simulink library "control_allocation_lib"  (R2018b)
settings: Solver=VariableStepAuto  StartTime=0.0  StopTime=10.0  RelTol=1e-3
undefined symbols (not defined in the file or in its folder): ca
libraries: $bdroot x1
settings Model: Creator=Ybeyer  LastModifiedBy=yannic
settings DebuggingCC: LibraryContextMissingDiagnostic=none
settings SFSimCC: SimUseLocalCustomCode=off
settings RTWCC: RTWUseLocalCustomCode=off
settings CodeAppCC: StateflowObjectComments=on

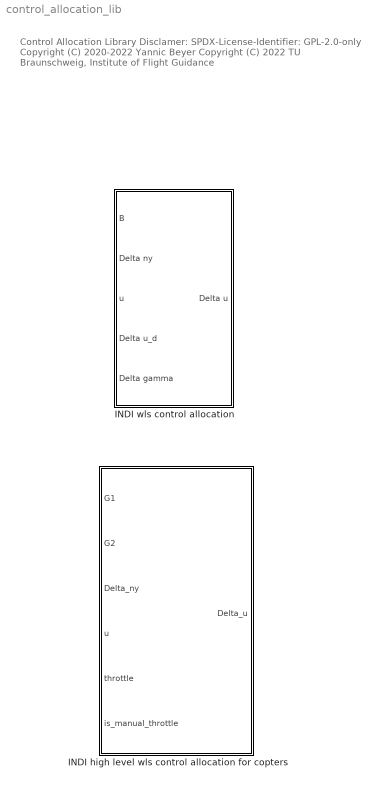
== system control_allocation_lib ==
  note: Control Allocation Library
      |
      | Disclamer:
      | SPDX-License-Identifier: GPL-2.0-only
      |
      | Copyright (C) 2020-2022 Yannic Beyer
      | Copyright (C) 2022 TU Braunschweig, Institute of Flight Guidance
  INDI high level wls control allocation for copters : Subsystem  mask{ca=ca}
      mask prompts: ca "control allocation parameters struct"
      mask DialogControl DescGroupVar Prompt: INDI high level control allocation
      mask DialogControl DescTextVar Prompt: It wraps the INDI control allocation block and adds some high level usability features.
      mask DialogControl Control2 Prompt: This block makes manual throttle control possible. Moreover, it not only considers the control effectiveness G1 but also the effectiveness of the control input derivative G2 [1].
      mask DialogControl Control3 Prompt: [1] Smeur, E. J., Chu, Q., & de Croon, G. C. (2016). Adaptive incremental nonlinear dynamic inversion for attitude control of micro air vehicles. Journal of Guidance, Control, and Dynamics, 39(3), 450-461.
      mask DialogControl Control4 Prompt: To load a control allocation parameters struct, see controlAllocationWlsLoadParams
  INDI wls control allocation : Subsystem  mask{ca=ca}
      mask prompts: ca "control allocation parameters struct"
      mask DialogControl DescGroupVar Prompt: INDI control allocation
      mask DialogControl DescTextVar Prompt: Solve wls control allocation algorithm for INDI.
      mask DialogControl Control2 Prompt: The control allocation algorithm is adjusted to INDI according to
      mask DialogControl Control3 Prompt: Smeur, E., Höppener, D., & Wagter, C. D. (2017). Prioritized Control Allocation for Quadrotors Subject to Saturation, In H. D. P. J.-M. Moschetta, G. Hattenberger (Ed.), International Micro Air Vehicle Conference and Flight Competition 2017 (pp. 37-43). Toulouse, France.
      mask DialogControl Control4 Prompt: To load a control allocation parameters struct, see controlAllocationWlsLoadParams

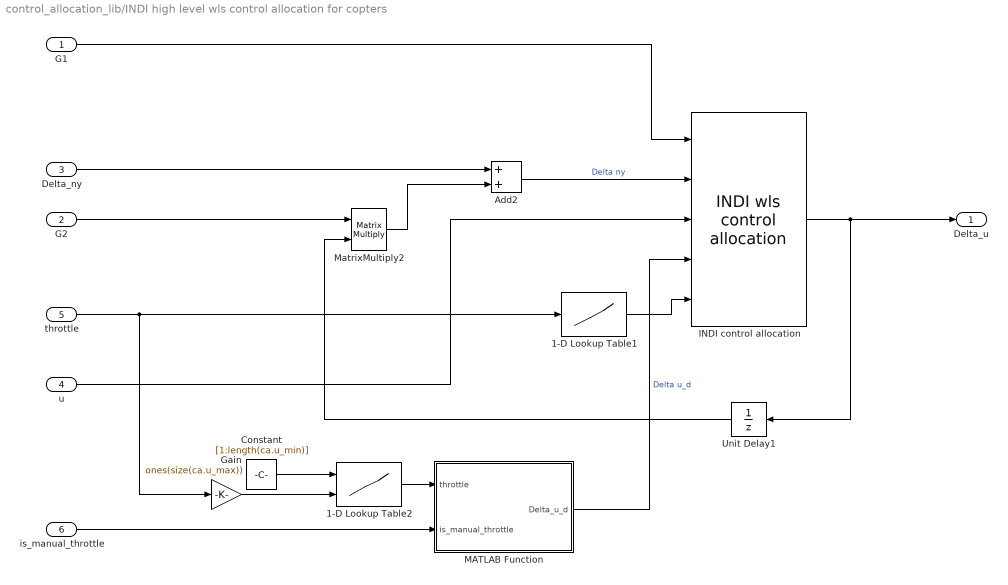
== system control_allocation_lib/INDI high level wls control allocation for copters ==
  G1 : Inport
  G2 : Inport  Port=2
  Delta_ny : Inport  Port=3
  u : Inport  Port=4
  throttle : Inport  Port=5
  is_manual_throttle : Inport  Port=6
  1-D Lookup Table1 : Lookup_n-D  NumberOfTableDimensions=1  BreakpointsForDimension1=[0,0.1,0.2,1]  Table=[-0.99999999*ca.gamma*[1,1],0,0]  InternalRulePriority=Speed  RndMeth=Simplest  InputSameDT=on
  1-D Lookup Table2 : Lookup_n-D  BreakpointsForDimension1=[1:length(ca.u_min)]'  BreakpointsForDimension2=[0,1]  Table=[ca.u_min,ca.u_max]  ExtrapMethod=Clip  InternalRulePriority=Speed  RndMeth=Simplest  InputSameDT=on
  Add2 : Sum
  Constant : Constant  Value=[1:length(ca.u_min)]  OutDataTypeStr=Inherit: Inherit via back propagation
  Gain : Gain  Gain=ones(size(ca.u_max))
  INDI control allocation : $bdroot/INDI wls control allocation  ca=ca
  MATLAB Function : MATLAB Function  TreatAsAtomicUnit=on
  MatrixMultiply2 : Product  Multiplication=Matrix(*)
  Unit Delay1 : UnitDelay  SampleTime=-1
  Delta_u : Outport
  wires:
  throttle/1 -> Gain/1, 1-D Lookup Table1/1
  G2/1 -> MatrixMultiply2/1
  MatrixMultiply2/1 -> Add2/2
  G1/1 -> INDI control allocation/1
  Add2/1 -> INDI control allocation/2  "Delta ny"
  u/1 -> INDI control allocation/3
  INDI control allocation/1 -> Delta_u/1, Unit Delay1/1
  1-D Lookup Table1/1 -> INDI control allocation/5
  Delta_ny/1 -> Add2/1
  Unit Delay1/1 -> MatrixMultiply2/2
  MATLAB Function/1(Delta_u_d) -> INDI control allocation/4  "Delta u_d"
  is_manual_throttle/1 -> MATLAB Function/2(is_manual_throttle)
  1-D Lookup Table2/1 -> MATLAB Function/1(throttle)
  Gain/1 -> 1-D Lookup Table2/2
  Constant/1 -> 1-D Lookup Table2/1

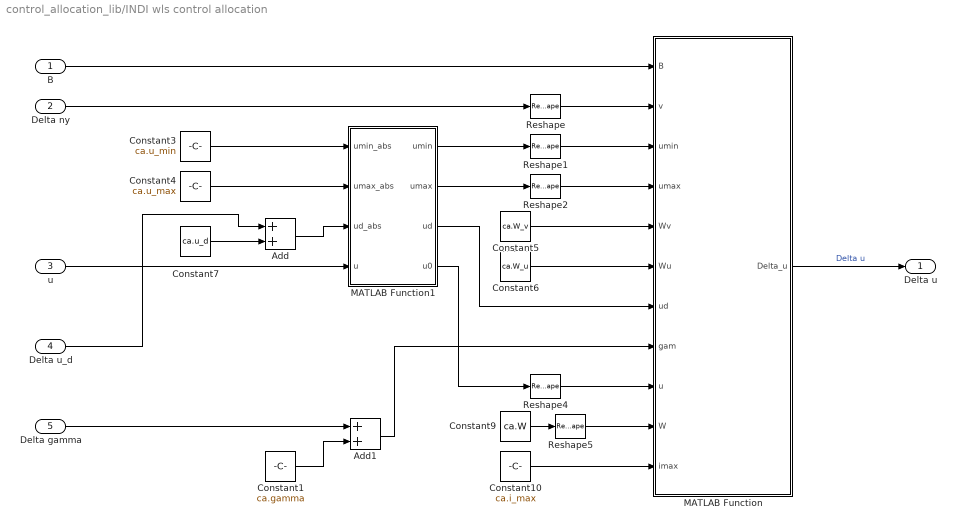
== system control_allocation_lib/INDI wls control allocation ==
  B : Inport
  Delta ny : Inport  Port=2
  u : Inport  Port=3
  Delta u_d : Inport  Port=4
  Delta gamma : Inport  Port=5
  Add : Sum  OutDataTypeStr=Inherit: Same as first input
  Add1 : Sum
  Constant1 : Constant  Value=ca.gamma
  Constant10 : Constant  Value=ca.i_max
  Constant3 : Constant  Value=ca.u_min
  Constant4 : Constant  Value=ca.u_max
  Constant5 : Constant  Value=ca.W_v
  Constant6 : Constant  Value=ca.W_u
  Constant7 : Constant  Value=ca.u_d
  Constant9 : Constant  Value=ca.W
  MATLAB Function : MATLAB Function  TreatAsAtomicUnit=on
  MATLAB Function1 : MATLAB Function  TreatAsAtomicUnit=on
  Reshape{,1..2,4..5} (5 alike) : Reshape  OutputDimensionality=Column vector (2-D)
  Delta u : Outport
  wires:
  Constant1/1 -> Add1/2
  Delta gamma/1 -> Add1/1
  Add1/1 -> MATLAB Function/8(gam)
  u/1 -> MATLAB Function1/4(u)
  MATLAB Function/1(Delta_u) -> Delta u/1  "Delta u"
  Constant10/1 -> MATLAB Function/11(imax)
  Constant7/1 -> Add/2
  Reshape5/1 -> MATLAB Function/10(W)
  Constant5/1 -> MATLAB Function/5(Wv)
  Delta u_d/1 -> Add/1
  Constant3/1 -> MATLAB Function1/1(umin_abs)
  MATLAB Function1/2(umax) -> Reshape2/1
  B/1 -> MATLAB Function/1(B)
  Delta ny/1 -> Reshape/1
  Constant4/1 -> MATLAB Function1/2(umax_abs)
  Reshape/1 -> MATLAB Function/2(v)
  Reshape2/1 -> MATLAB Function/4(umax)
  Constant6/1 -> MATLAB Function/6(Wu)
  Reshape1/1 -> MATLAB Function/3(umin)
  Constant9/1 -> Reshape5/1
  MATLAB Function1/1(umin) -> Reshape1/1
  MATLAB Function1/4(u0) -> Reshape4/1
  Reshape4/1 -> MATLAB Function/9(u)
  MATLAB Function1/3(ud) -> MATLAB Function/7(ud)
  Add/1 -> MATLAB Function1/3(ud_abs)

== matlab function control_allocation_lib/INDI high level wls control allocation for copters/MATLAB Function ==
  data: throttle input; Delta_u_d output; is_manual_throttle input
function Delta_u_d = fcn(throttle, is_manual_throttle)
Delta_u_d = zeros(size(is_manual_throttle));
Delta_u_d(is_manual_throttle) = throttle(is_manual_throttle);
end

== matlab function control_allocation_lib/INDI wls control allocation/MATLAB Function ==
  data: B input; v input; umin input; umax input; Wv input; Wu input; ud input; gam input; u input; Delta_u output; W input; imax input
function Delta_u = fcn(B,v,umin,umax,Wv,Wu,ud,gam,u,W,imax)

[Delta_u,~,~] = wls_alloc(B,v,umin,umax,Wv,Wu,ud,gam,u,W,imax);

end

== matlab function control_allocation_lib/INDI wls control allocation/MATLAB Function1 ==
  data: umin_abs input; umax_abs input; ud_abs input; u input; umin output; umax output; ud output; u0 output
function [umin,umax,ud,u0] = fcn(umin_abs,umax_abs,ud_abs,u)

umin = umin_abs - u;
umax = umax_abs - u;
ud = ud_abs - u;
u0 = 0.5 * (umin+umax);

end
